simulink library "targets_stateflow_algorithms"  (Simulink 7.6)
settings: Solver=ode45  SolverMode=SingleTasking  StartTime=0.0  StopTime=10.0  RelTol=1e-3
values from neighbouring files (symbols this model uses):
  A1 = [1 -0.740818220682]    [targets_fsysdat.mat]
  A2 = [1 -0.740818220682]    [targets_fsysdat.mat]
  B1 = [8.76963147833 -8.51044969901]    [targets_fsysdat.mat]
  B2 = [0 0.259181779318]    [targets_fsysdat.mat]
  DISABLED = 3    [targets_fsysdat.mat]
  hys = 25    [targets_fsysdat.mat]
  Ki = 0.012    [targets_fsysdat.mat]
  LOW = 1    [targets_fsysdat.mat]
  max_ego = 1.2    [targets_fsysdat.mat]
  max_press = 1    [targets_fsysdat.mat]
  max_speed = 628    [targets_fsysdat.mat]
  max_throt = 90    [targets_fsysdat.mat]
  min_press = 0.0078    [targets_fsysdat.mat]
  min_throt = 3    [targets_fsysdat.mat]
  press = [0.05 0.1 0.15 0.2 0.25 0.3 0.35 0.4 0.45 0.5 0.55 0.6 ... (19 elements, 1x19)]    [targets_fsysdat.mat]
  PressEst = [0.806253176324 0.553142316929 0.37151500209 0.277667903103 0.220198954207 0.181288665766 0.153200000489 0.115431020872 0.0913067476324 0.0746519188607 0.0625231108324 0.0533383634277 ... (306 elements, 18x17)]    [targets_fsysdat.mat]
  pumpCon = [-0.0556348 -0.0022828 0.0256932 0.0435188 0.0562692 0.0661194857143 0.0741572 0.08697 0.0972452 0.106070342857 0.1139892 0.121303866667 ... (342 elements, 18x19)]    [targets_fsysdat.mat]
  RICH = 2    [targets_fsysdat.mat]
  SpeedEst = [471.837839721 550.80940091 777.559313277 1080.9243499 1418.36795322 1769.7468768 2125.37309264 2480.20345067 2831.37796793 3177.14006959 3516.32917143 4064.90417867 ... (323 elements, 17x19)]    [targets_fsysdat.mat]
  ThrotEst = [0 0 0 0 0 0 0 0 0 0 0 0 ... (342 elements, 18x19)]    [targets_fsysdat.mat]
  zero_thresh = 250    [targets_fsysdat.mat]
undefined symbols (not defined in the file or in its folder): fixpt_evenspace_cleanup
libraries: simulink x2, fixpt_lib_4 x1
settings Model: Creator=The MathWorks Inc.

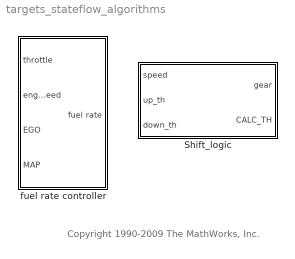
== system targets_stateflow_algorithms ==
  note: Copyright 1990-2009 The MathWorks, Inc.
  Shift_logic : Stateflow chart  TreatAsAtomicUnit=on
  fuel rate controller : Subsystem

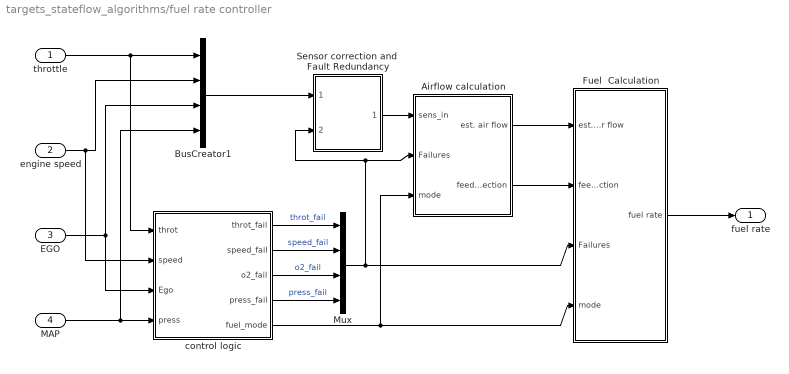
== system targets_stateflow_algorithms/fuel rate controller ==
  throttle : Inport
  engine speed : Inport  Port=2
  EGO : Inport  Port=3
  MAP : Inport  Port=4
  Airflow calculation : Subsystem
  BusCreator1 : BusCreator
  Fuel  Calculation : Subsystem
  Mux : Mux
  Sensor correction and  Fault Redundancy : Subsystem
  control logic : Stateflow chart  Description=Stateflow diagram to determine control system operating mode  TreatAsAtomicUnit=on
  fuel rate : Outport  InitialOutput=0
  wires:
  control logic/4(press_fail) -> Mux/4  "press_fail"
  control logic/3(o2_fail) -> Mux/3  "o2_fail"
  control logic/2(speed_fail) -> Mux/2  "speed_fail"
  control logic/1(throt_fail) -> Mux/1  "throt_fail"
  Mux/1 -> Fuel  Calculation/3(Failures), Airflow calculation/2(Failures), Sensor correction and  Fault Redundancy/2(Failures)
  Sensor correction and  Fault Redundancy/1(Corrected) -> Airflow calculation/1(sens_in)
  Airflow calculation/1(est. air flow) -> Fuel  Calculation/1(est. air flow)
  Fuel  Calculation/1(fuel rate) -> fuel rate/1
  Airflow calculation/2(feedback correction) -> Fuel  Calculation/2(feedback correction)
  control logic/5(fuel_mode) -> Fuel  Calculation/4(mode), Airflow calculation/3(mode)
  BusCreator1/1 -> Sensor correction and  Fault Redundancy/1(Sensors)
  throttle/1 -> control logic/1(throt), BusCreator1/1
  engine speed/1 -> control logic/2(speed), BusCreator1/2
  EGO/1 -> control logic/3(Ego), BusCreator1/3
  MAP/1 -> control logic/4(press), BusCreator1/4

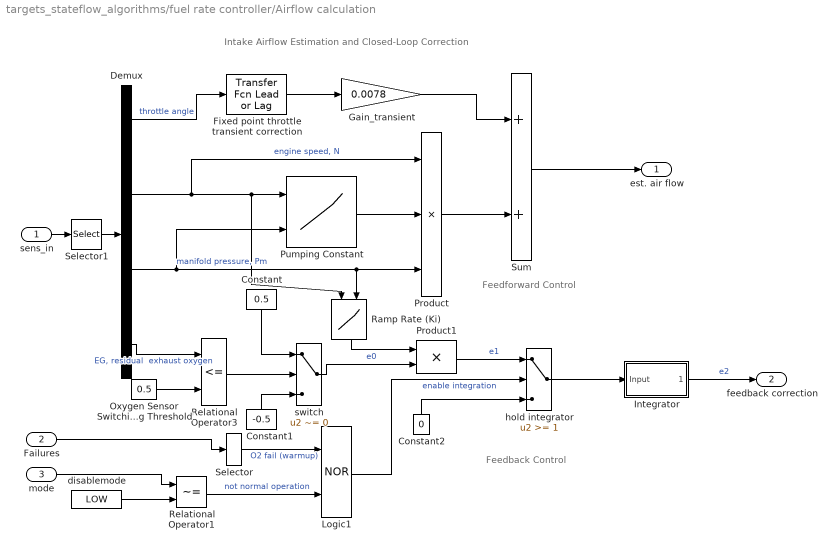
== system targets_stateflow_algorithms/fuel rate controller/Airflow calculation ==
  note: Feedforward Control
  note: Feedback Control
  note: Intake Airflow Estimation and Closed-Loop Correction
  sens_in : Inport
  Failures : Inport  Port=2
  mode : Inport  Port=3
  Constant : Constant  Value=0.5  OutDataTypeStr=fixdt(1,16,8)
  Constant1 : Constant  Value=-0.5  OutDataTypeStr=Inherit: Inherit via back propagation
  Constant2 : Constant  Value=0  OutDataTypeStr=Inherit: Inherit via back propagation
  Demux : Demux
  Fixed point throttle transient correction : simulink/Discrete/Transfer Fcn Lead or Lag  SystemSampleTime=-1  PoleZ=0.8  ZeroZ=1  ICPrevOutput=0.0  ICPrevInput=0.0  DoSatur=off
  Gain_transient : Gain  Gain=0.0078  OutDataTypeStr=fixdt(1,16,8)  SaturateOnIntegerOverflow=on  ParamDataTypeStr=Inherit: Same as input
  Integrator : Subsystem  Description=REQ: PM=30deg, GM=6db
      mask Display: disp('T/(Z-1)')
  Logic1 : Logic  Operator=NOR
  Oxygen Sensor Switching Threshold : Constant  Value=0.5  OutDataTypeStr=Inherit: Inherit via back propagation
  Product : Product  Inputs=3  OutDataTypeStr=fixdt(1,16,8)  SaturateOnIntegerOverflow=on
  Product1 : Product  SaturateOnIntegerOverflow=on  InputSameDT=on  OutDataTypeStr=Inherit: Same as first input
  Pumping Constant : Lookup2D  RowIndex=SpeedVect  ColumnIndex=fixpt_evenspace_cleanup(press,sfix(16),2^-14)  Table=pumpCon  LookUpMeth=Interpolation-Use End Values  OutDataTypeStr=fixdt(1,16,16)  SaturateOnIntegerOverflow=on
  Ramp Rate (Ki) : Lookup2D  RowIndex=[100:100:500]  ColumnIndex=fixpt_evenspace_cleanup([0:0.2:1],sfix(16),2^-14)  Table=[1:5]'*[1:6]*Ki  LookUpMeth=Interpolation-Use End Values  OutDataTypeStr=fixdt(1,16,8)  SaturateOnIntegerOverflow=on
  Relational Operator1 : RelationalOperator  Operator=~=  InputSameDT=on
  Relational Operator3 : RelationalOperator  Operator=<=  InputSameDT=on
  Selector : Selector  InputPortWidth=4  IndexOptions=Index vector (dialog)  Indices=3  OutputSizes=1
  Selector1 : Selector  InputPortWidth=4  IndexOptions=Index vector (dialog)  Indices=[1 2 4 3]  OutputSizes=1
  Sum : Sum  Inputs=2  SaturateOnIntegerOverflow=on  InputSameDT=on  OutDataTypeStr=Inherit: Same as first input
  disablemode : Constant  Value=LOW
  hold integrator : Switch  Threshold=1  SaturateOnIntegerOverflow=on  InputSameDT=on
  switch : Switch  Criteria=u2 ~= 0  Threshold=1  OutDataTypeStr=Inherit: Inherit via back propagation  SaturateOnIntegerOverflow=on  InputSameDT=on
  est. air flow : Outport  InitialOutput=0
  feedback correction : Outport  Port=2  InitialOutput=0
  wires:
  Gain_transient/1 -> Sum/1
  Fixed point throttle transient correction/1 -> Gain_transient/1
  Integrator/1(Output) -> feedback correction/1  "e2"
  Sum/1 -> est. air flow/1
  Constant1/1 -> switch/3
  Relational Operator3/1 -> switch/2
  switch/1 -> Product1/2  "e0"
  Logic1/1 -> hold integrator/2  "enable integration"
  hold integrator/1 -> Integrator/1(Input)
  Product1/1 -> hold integrator/1  "e1"
  Constant2/1 -> hold integrator/3
  Ramp Rate (Ki)/1 -> Product1/1
  Constant/1 -> switch/1
  Oxygen Sensor Switching Threshold/1 -> Relational Operator3/2
  Demux/4 -> Relational Operator3/1  "EG, residual  exhaust oxygen"
  Relational Operator1/1 -> Logic1/2  "not normal operation"
  disablemode/1 -> Relational Operator1/2
  Failures/1 -> Selector/1
  Selector/1 -> Logic1/1  "O2 fail (warmup)"
  Demux/1 -> Fixed point throttle transient correction/1  "throttle angle"
  Selector1/1 -> Demux/1
  Demux/2 -> Product/1, Ramp Rate (Ki)/1, Pumping Constant/1  "engine speed, N"
  Demux/3 -> Pumping Constant/2, Product/3, Ramp Rate (Ki)/2  "manifold pressure, Pm"
  Product/1 -> Sum/2
  Pumping Constant/1 -> Product/2
  sens_in/1 -> Selector1/1
  mode/1 -> Relational Operator1/1

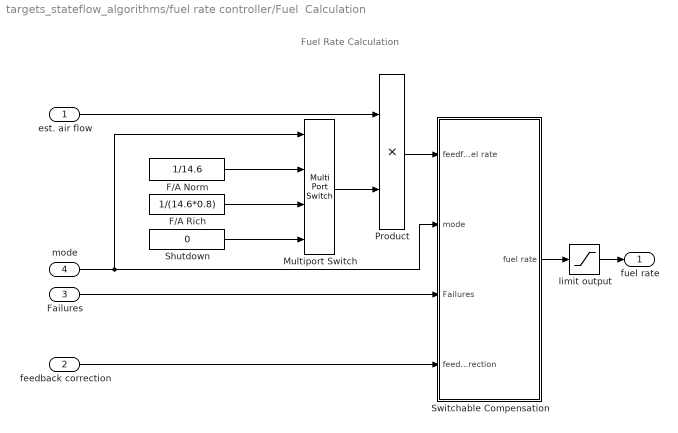
== system targets_stateflow_algorithms/fuel rate controller/Fuel  Calculation ==
  note: Fuel Rate Calculation
  est. air flow : Inport
  feedback correction : Inport  Port=2
  Failures : Inport  Port=3
  mode : Inport  Port=4
  F/A Norm : Constant  Value=1/14.6  OutDataTypeStr=fixdt(1,16,8)
  F/A Rich : Constant  Value=1/(14.6*0.8)  OutDataTypeStr=Inherit: Inherit via back propagation
  Multiport Switch : MultiPortSwitch  zeroidx=off  SaturateOnIntegerOverflow=on  InputSameDT=on
  Product : Product  OutDataTypeStr=fixdt(1,16,12)  SaturateOnIntegerOverflow=on  InputSameDT=on
  Shutdown : Constant  Value=0  OutDataTypeStr=Inherit: Inherit via back propagation
  Switchable Compensation : Subsystem
  limit output : Saturate  UpperLimit=100  LowerLimit=0
  fuel rate : Outport  InitialOutput=0
  wires:
  Switchable Compensation/1(fuel rate) -> limit output/1
  Product/1 -> Switchable Compensation/1(feedforward fuel rate)
  Failures/1 -> Switchable Compensation/3(Failures)
  mode/1 -> Multiport Switch/1, Switchable Compensation/2(mode)
  Multiport Switch/1 -> Product/2
  est. air flow/1 -> Product/1
  F/A Norm/1 -> Multiport Switch/2
  F/A Rich/1 -> Multiport Switch/3
  Shutdown/1 -> Multiport Switch/4
  feedback correction/1 -> Switchable Compensation/4(feedback correction)
  limit output/1 -> fuel rate/1

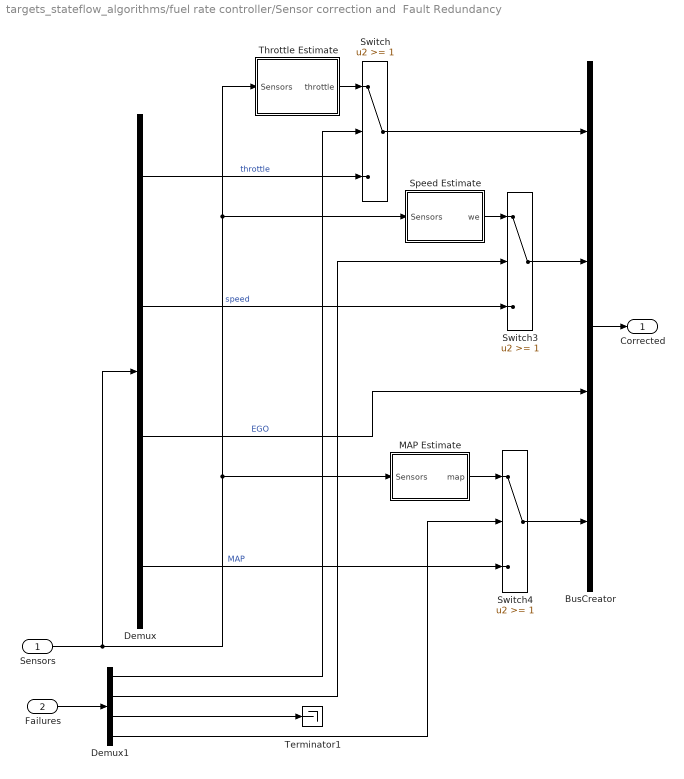
== system targets_stateflow_algorithms/fuel rate controller/Sensor correction and  Fault Redundancy ==
  Sensors : Inport
  Failures : Inport  Port=2
  BusCreator : BusCreator
  Demux : Demux
  Demux1 : Demux
  MAP Estimate : Subsystem  TreatAsAtomicUnit=on
  Speed Estimate : Subsystem  TreatAsAtomicUnit=on
  Switch : Switch  Threshold=1  SaturateOnIntegerOverflow=on  InputSameDT=on
  Switch3 : Switch  Threshold=1  SaturateOnIntegerOverflow=on  InputSameDT=on
  Switch4 : Switch  Threshold=1  SaturateOnIntegerOverflow=on
  Terminator1 : Terminator
  Throttle Estimate : Subsystem  TreatAsAtomicUnit=on
  Corrected : Outport  InitialOutput=0
  wires:
  BusCreator/1 -> Corrected/1
  Demux/3 -> BusCreator/3  "EGO"
  Switch/1 -> BusCreator/1
  Failures/1 -> Demux1/1
  Demux/1 -> Switch/3  "throttle"
  Throttle Estimate/1(throttle) -> Switch/1
  Demux1/3 -> Terminator1/1
  Demux1/1 -> Switch/2
  Switch3/1 -> BusCreator/2
  Demux/2 -> Switch3/3  "speed"
  Speed Estimate/1(we) -> Switch3/1
  Demux1/2 -> Switch3/2
  Demux1/4 -> Switch4/2
  Switch4/1 -> BusCreator/4
  Demux/4 -> Switch4/3  "MAP"
  MAP Estimate/1(map) -> Switch4/1
  Sensors/1 -> MAP Estimate/1(Sensors), Speed Estimate/1(Sensors), Throttle Estimate/1(Sensors), Demux/1

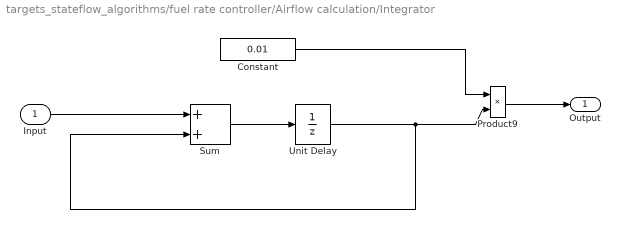
== system targets_stateflow_algorithms/fuel rate controller/Airflow calculation/Integrator ==
  Input : Inport
  Constant : Constant  Value=0.01  OutDataTypeStr=fixdt(1,16,12)
  Product9 : Product  SaturateOnIntegerOverflow=on  OutDataTypeStr=Inherit: Same as first input
  Sum : Sum  Tag=S16 2^-10  SaturateOnIntegerOverflow=on  InputSameDT=on  LockScale=on
  Unit Delay : UnitDelay  X0=-1  SampleTime=0.01
  Output : Outport
  wires:
  Input/1 -> Sum/1
  Sum/1 -> Unit Delay/1
  Product9/1 -> Output/1
  Constant/1 -> Product9/1
  Unit Delay/1 -> Sum/2, Product9/2

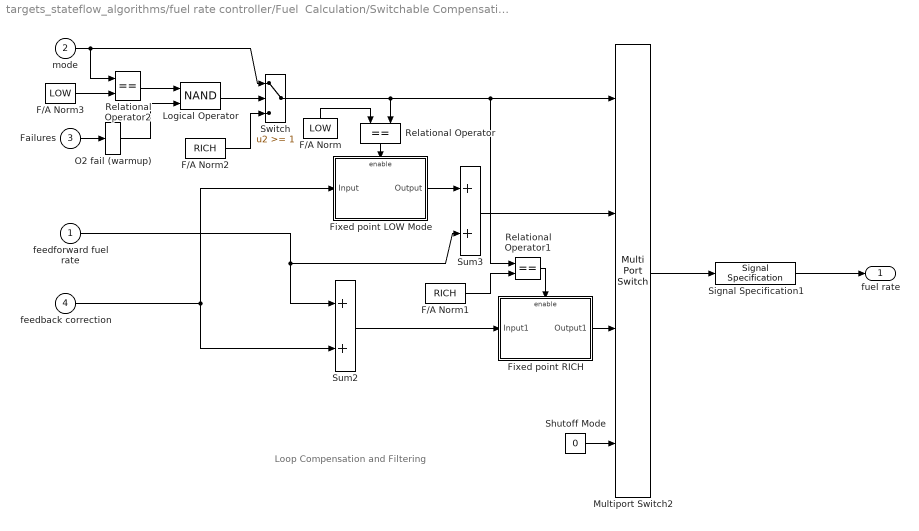
== system targets_stateflow_algorithms/fuel rate controller/Fuel  Calculation/Switchable Compensation ==
  note: Loop Compensation and Filtering
  feedforward fuel rate : Inport
  mode : Inport  Port=2
  Failures : Inport  Port=3
  feedback correction : Inport  Port=4
  F/A Norm : Constant  Value=LOW
  F/A Norm1 : Constant  Value=RICH
  F/A Norm2 : Constant  Value=RICH
  F/A Norm3 : Constant  Value=LOW
  Fixed point LOW Mode : Subsystem  TreatAsAtomicUnit=on  mask(enabled discrete-time transfer function){num=B1, den=A1, u0=-0.01, y0=-0.01, Ts=0.01}
      mask prompts: num "numerator polynomial"; den "denominator polynomial"; u0 "initial input"; y0 "initial output"; Ts "sample time"
      mask Display: dpoly(num,den,'z')
  Fixed point RICH : Subsystem  TreatAsAtomicUnit=on  mask(enabled discrete-time transfer function){num=B2, den=A2, u0=1.6, y0=1.6, Ts=0.01}
      mask prompts: num "numerator polynomial"; den "denominator polynomial"; u0 "initial input"; y0 "initial output"; Ts "sample time"
      mask Display: dpoly(num,den,'z')
  Logical Operator : Logic  Operator=NAND
  Multiport Switch2 : MultiPortSwitch  zeroidx=off  SaturateOnIntegerOverflow=on  InputSameDT=on
  O2 fail (warmup) : Selector  InputPortWidth=4  IndexOptions=Index vector (dialog)  Indices=3  OutputSizes=1
  Relational Operator : RelationalOperator  Operator===  InputSameDT=on
  Relational Operator1 : RelationalOperator  Operator===  InputSameDT=on
  Relational Operator2 : RelationalOperator  Operator===  InputSameDT=on
  Shutoff Mode : Constant  Value=0  OutDataTypeStr=Inherit: Inherit via back propagation
  Signal Specification1 : SignalSpecification  SampleTime=0.01
  Sum2 : Sum  OutDataTypeStr=fixdt(1,16,8)  SaturateOnIntegerOverflow=on  InputSameDT=on
  Sum3 : Sum  SaturateOnIntegerOverflow=on  OutDataTypeStr=Inherit: Same as first input
  Switch : Switch  Threshold=1  SaturateOnIntegerOverflow=on  InputSameDT=on
  fuel rate : Outport  InitialOutput=0
  wires:
  Fixed point LOW Mode/1(Output) -> Sum3/1
  Fixed point RICH/1(Output1) -> Multiport Switch2/3
  Signal Specification1/1 -> fuel rate/1
  O2 fail (warmup)/1 -> Logical Operator/2
  Failures/1 -> O2 fail (warmup)/1
  Relational Operator2/1 -> Logical Operator/1
  F/A Norm3/1 -> Relational Operator2/2
  mode/1 -> Relational Operator2/1, Switch/1
  Logical Operator/1 -> Switch/2
  F/A Norm2/1 -> Switch/3
  F/A Norm/1 -> Relational Operator/1
  Switch/1 -> Relational Operator/2, Multiport Switch2/1, Relational Operator1/1
  Multiport Switch2/1 -> Signal Specification1/1
  Relational Operator/1 -> Fixed point LOW Mode/Enable
  Relational Operator1/1 -> Fixed point RICH/Enable
  F/A Norm1/1 -> Relational Operator1/2
  Shutoff Mode/1 -> Multiport Switch2/4
  Sum2/1 -> Fixed point RICH/1(Input1)
  Sum3/1 -> Multiport Switch2/2
  feedback correction/1 -> Fixed point LOW Mode/1(Input), Sum2/2
  feedforward fuel rate/1 -> Sum2/1, Sum3/2

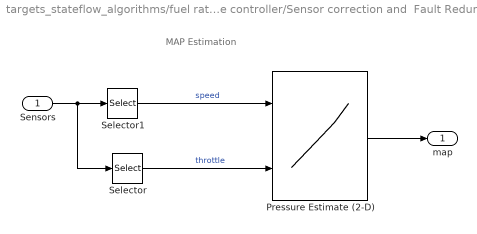
== system targets_stateflow_algorithms/fuel rate controller/Sensor correction and  Fault Redundancy/MAP Estimate ==
  note: MAP Estimation
  Sensors : Inport
  Pressure Estimate (2-D) : Lookup2D  RowIndex=SpeedVect  ColumnIndex=ThrotVect  Table=PressEst  LookUpMeth=Interpolation-Use End Values  OutDataTypeStr=fixdt(1,16,14)  SaturateOnIntegerOverflow=on
  Selector : Selector  InputPortWidth=4  IndexOptions=Index vector (dialog)  Indices=1  OutputSizes=1
  Selector1 : Selector  InputPortWidth=4  IndexOptions=Index vector (dialog)  Indices=2  OutputSizes=1
  map : Outport  InitialOutput=0
  wires:
  Pressure Estimate (2-D)/1 -> map/1
  Selector/1 -> Pressure Estimate (2-D)/2  "throttle"
  Selector1/1 -> Pressure Estimate (2-D)/1  "speed"
  Sensors/1 -> Selector/1, Selector1/1

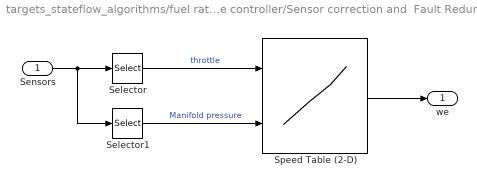
== system targets_stateflow_algorithms/fuel rate controller/Sensor correction and  Fault Redundancy/Speed Estimate ==
  Sensors : Inport
  Selector : Selector  InputPortWidth=4  IndexOptions=Index vector (dialog)  Indices=1  OutputSizes=1
  Selector1 : Selector  InputPortWidth=4  IndexOptions=Index vector (dialog)  Indices=4  OutputSizes=1
  Speed Table (2-D) : Lookup2D  RowIndex=ThrotVect  ColumnIndex=fixpt_evenspace_cleanup(press,sfix(16),2^-14)  Table=SpeedEst  LookUpMeth=Interpolation-Use End Values  OutDataTypeStr=fixdt(1,16,1)  SaturateOnIntegerOverflow=on
  we : Outport  InitialOutput=0
  wires:
  Selector1/1 -> Speed Table (2-D)/2  "Manifold pressure"
  Selector/1 -> Speed Table (2-D)/1  "throttle"
  Sensors/1 -> Selector/1, Selector1/1
  Speed Table (2-D)/1 -> we/1

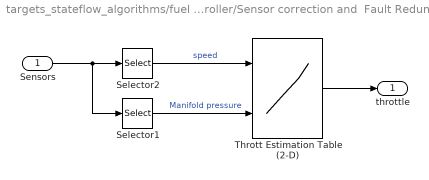
== system targets_stateflow_algorithms/fuel rate controller/Sensor correction and  Fault Redundancy/Throttle Estimate ==
  Sensors : Inport
  Selector1 : Selector  InputPortWidth=4  IndexOptions=Index vector (dialog)  Indices=4  OutputSizes=1
  Selector2 : Selector  InputPortWidth=4  IndexOptions=Index vector (dialog)  Indices=2  OutputSizes=1
  Thrott Estimation Table (2-D) : Lookup2D  RowIndex=SpeedVect  ColumnIndex=fixpt_evenspace_cleanup(press,sfix(16),2^-14)  Table=ThrotEst  LookUpMeth=Interpolation-Use End Values  OutDataTypeStr=fixdt(1,16,5)  SaturateOnIntegerOverflow=on
  throttle : Outport  InitialOutput=0
  wires:
  Thrott Estimation Table (2-D)/1 -> throttle/1
  Selector1/1 -> Thrott Estimation Table (2-D)/2  "Manifold pressure"
  Selector2/1 -> Thrott Estimation Table (2-D)/1  "speed"
  Sensors/1 -> Selector1/1, Selector2/1

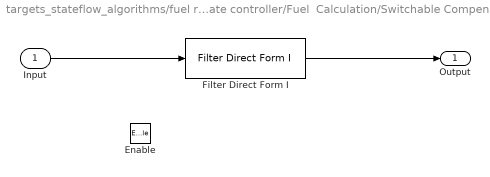
== system targets_stateflow_algorithms/fuel rate controller/Fuel  Calculation/Switchable Compensation/Fixed point LOW Mode ==
  Input : Inport
  Enable : EnablePort  StatesWhenEnabling=reset
  Filter Direct Form I : fixpt_lib_4/Filters/Filter Direct Form I  SystemSampleTime=-1  NumCoefVec=B1  DenCoefVec=A1(2)  ICPrevOutput=0.0  ICPrevInput=0.0  DoSatur=off
  Output : Outport
  wires:
  Filter Direct Form I/1 -> Output/1
  Input/1 -> Filter Direct Form I/1

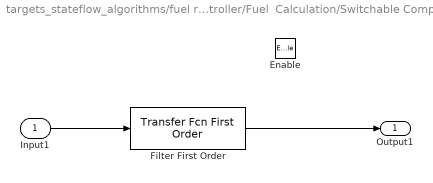
== system targets_stateflow_algorithms/fuel rate controller/Fuel  Calculation/Switchable Compensation/Fixed point RICH ==
  Input1 : Inport
  Enable : EnablePort  StatesWhenEnabling=reset
  Filter First Order : simulink/Discrete/Transfer Fcn First Order  SystemSampleTime=-1  PoleZ=-den(2)  ICPrevOutput=y0  DoSatur=off
  Output1 : Outport
  wires:
  Filter First Order/1 -> Output1/1
  Input1/1 -> Filter First Order/1

== stateflow chart fuel rate controller/control logic ==
  settings: updateMethod=DISCRETE  sampleTime=0.01
  state O2 [parallel]
    settings: executionOrder=1  description=This state determines the validity of the exhaust gas oxygen sensor (EGO) data.
    state fail
      entry: o2_fail = 1;
      settings: description=The EGO sensor has failed.
    state warmup
      entry: o2_fail = 1;
      during: warmup_clk++;
      settings: description=The EGO sensor must come up to temperature before its data is reliable.
    state normal
      entry: o2_fail = 0;
      settings: description=Normal EGO sensor operation gives a reliable indication of excess oxygen in the exhaust gas, from which air/fuel mixture can be inferred.
    O2.fail -> O2.normal : [Ego < max_ego] /
        | Fail.DEC
    O2.normal -> O2.fail : [Ego > max_ego]/
        | Fail.INC
      settings: description=The failure condition is indicated by excessive output voltage.
    (default) -> warmup
    warmup -> O2.normal : [warmup_clk>480]
      settings: description=It is assumed that the time o2_t_thresh is sufficient for the sensor to warm up to operational temperature.
  state Pressure [parallel]
    settings: executionOrder=2  description=This state assesses the validity of the manifold absolute pressure (MAP) sensor.
    state press_norm
      entry:  press_fail = 0;
      settings: description=The manifold pressure sensor gives a reliable indication of absolute pressure (MAP).
    state press_fail
      entry: press_fail = 1;
      settings: description=The pressure sensor (manifold, or MAP) no longer produces reliable data.
    press_norm -> press_fail : [press > max_press | press < min_press]
        | /Fail.INC
    (default) -> press_norm
    press_fail -> press_norm : [press > min_press & press < max_press] /
        | Fail.DEC
  state Throttle [parallel]
    settings: executionOrder=3  description=This state determines the validity of the throttle sensor signal.
    state normal
      entry: throt_fail = 0;
      settings: description=The throttle sensor gives a reliable indication of the angle of the throttle plate.
    state fail
      entry: throt_fail = 1;
      settings: description=Signal levels indicate that the throttle sensor data is no longer valid.
    Throttle.normal -> Throttle.fail : [throt> max_throt | throt < min_throt]/
        | Fail.INC
      settings: description=A failure is indicated by data which is outside the expected range, typically due to an open or short circuit.
    (default) -> Throttle.normal
    Throttle.fail -> Throttle.normal : [throt >  min_throt & throt < max_throt]
        | / Fail.DEC
  state Speed [parallel]
    settings: executionOrder=4  description="This state infers the validity of the speed sensor data.  A failure is indicated by the presence of manifold vacuum at zero speed."
    state normal
      entry: speed_fail = 0;
      settings: description=The speed sensor data accurately represents the engine speed.
    state fail
      entry: speed_fail = 1;
      settings: description=The engine speed data is no longer available.
    Speed.normal -> Speed.fail : [speed==0 & press < zero_thresh]/
        | Fail.INC
      settings: description="Loss of a reliable speed sensor signal will indicate zero speed.  This is deemed invalid when the manifold vacuum indicates otherwise."
    (default) -> Speed.normal
    Speed.fail -> Speed.normal : [speed > 0] /
        | Fail.DEC
  state Fail [parallel]
    settings: executionOrder=5  description=This state maintains a count of the number of sensors in failure mode.
    state Multi
      settings: description=This state represents any of the conditions in which more than one sensor is in failure mode.
      state Three
        settings: description=Three of the engine sensors have failed.
      state Four
        settings: description=All four of the engine sensors have failed.
      state Two
        settings: description=Two of the engine sensors have failed.
      Three -> Four [order 1] : INC
      Two -> Three [order 2] : INC
      Four -> Three : DEC
      Three -> Two [order 2] : DEC
    state One
      settings: description=One of the engine sensors has failed.
    state None
      settings: description=Zero failures; all sensors are operational.
    (default) -> None
    None -> One : INC
    One -> Two [order 1] : INC
    Two -> One [order 1] : DEC
    One -> None [order 2] : DEC
  state Fueling_Mode [parallel]
    settings: executionOrder=6  description=This state interprets the other states in the chart to directly control the fueling mode.
    state Fuel_Disabled
      entry: fuel_mode = DISABLED;
      settings: description=The fuel is completely shut off while in this state.
      state Overspeed
        settings: description=The speed is dangerously high, so shut off the fuel.
      state Shutdown
        settings: description=Cut off system operation due to multiple sensor failures.
      Overspeed -> (junction 35) : [in(Speed.normal) & ...
          | speed < (max_speed - hys)]
      (junction 35) -> Shutdown [order 2] : [in(Fail.Multi)]
    state Running
      settings: description=The fuel is actively controlled while in this state.
      (history)
      state Low_Emissions
        entry: fuel_mode = LOW;
        (history)
        state Normal
          settings: description=All sensors are in correct operating modes, so effective closed-loop mixture control can be used.
        state Warmup
          settings: description="The sensors are all operational, but the oxygen (EGO) sensor is warming up.  We'll target a stoichiometric ratio, nonetheless, but won't close the loop around exhaust gas oxygen."
        (junction 36) -> Normal [order 2]
        Warmup -> (junction 36) : [in(O2.normal)]
      state Rich_Mixture
        entry: fuel_mode = RICH;
        settings: description=This mode enriches the mixture, lowering the air/fuel ratio.
        state Single_Failure
          settings: description=Continue uninterrupted engine operation, but with a richer mixture.
      Normal -> Single_Failure : [in(Fail.One)]
      Single_Failure -> Normal : [in(Fail.None)]
      (junction 36) -> Single_Failure [order 1] : [in(Fail.One)]
    Running -> Overspeed [order 2] : [ speed > max_speed ]
    (junction 35) -> Running [order 1] : [!in(Fail.Multi)]
    Running -> Shutdown [order 1] : enter(Fail.Multi)
    Shutdown -> Rich_Mixture : exit(Fail.Multi)
    (default) -> Warmup
  data: throt_fail output boolean; speed_fail output boolean; o2_fail output boolean; press_fail output boolean; throt input fixdt(1,16,5) [0..120]; speed input fixdt(1,16,1) [0..1000]; Ego input fixdt(1,16,7) [-5..12]; press input fixdt(1,16,7) [0..2]; fuel_mode output uint8 [1..3] =1; max_ego parameter fixdt(1,16,7) [0..12]; max_press parameter fixdt(1,16,7) [0..2]; min_press parameter fixdt(1,16,7) [0..2]; min_throt parameter fixdt(1,16,5) [0..120]; max_throt parameter fixdt(1,16,5) [0..120]; zero_thresh parameter fixdt(1,16,6) [0..500]; max_speed parameter fixdt(1,16,1) [0..1000]; hys parameter fixdt(1,16,5) [0..1000]; LOW parameter uint8; RICH parameter uint8; DISABLED parameter uint8; warmup_clk local uint16
  data throt settings: description=throttle plate angle
  data speed settings: description=engine angular velocity
  data Ego settings: description=Exhaust Gas Oxygen
  data press settings: description=Manifold Absolute Pressure (MAP)
  data fuel_mode settings: description=fuel control mode: LOW = stoichiometric mixture, RICH = rich mixture, DISABLED = shut down
  data max_ego settings: description=parameter represents the upper end of the EGO sensor range
  data max_press settings: description=parameter represents the upper limt of valid pressure readings
  data min_press settings: description=parameter for the lower end of the valid pressure sensor range
  data min_throt settings: description=minimum valid throttle angle
  data max_throt settings: description=parameter to indicate the maximum valid throttle angle reading
  data zero_thresh settings: description=minimum manifold pressure expected at zero speed
  data max_speed settings: description=parameter for the upper end of the safe engine speed range
  data hys settings: description=Hysteresis in the upper speed limit to avoid chatter at the threshold.
  data LOW settings: description="constant represents \"low emissions\" or stoichiometric fuel mixture mode"
  data RICH settings: description=constant represents rich fuel mixture mode
  data DISABLED settings: description=constant represents zero fuel mode
  events: DEC local EITHER_EDGE_EVENT; INC local EITHER_EDGE_EVENT

== stateflow chart Shift_logic ==
  settings: updateMethod=DISCRETE  sampleTime=0.04
  state gear_state [parallel]
    settings: executionOrder=1
    state fourth
      entry: gear = 4;
    state second
      entry: gear = 2;
    state third
      entry: gear = 3;
    state first
      entry: gear = 1;
    third -> fourth [order 1] : UP
    second -> third [order 1] : UP
    first -> second : UP
    (default) -> first
    fourth -> third : DOWN
    third -> second [order 2] : DOWN
    second -> first [order 2] : DOWN
  state selection_state [parallel]
    during: CALC_TH;
    settings: executionOrder=2
    state downshifting
    state upshifting
    state steady_state
    (default) -> steady_state
    steady_state -> upshifting [order 1] : [speed > up_th]
    steady_state -> downshifting [order 2] : [speed < down_th]
    upshifting -> steady_state [order 2] : [speed < up_th]
    downshifting -> steady_state [order 2] : [speed > down_th]
    downshifting -> steady_state [order 1] : after(TWAIT,tick)
        | [speed <= down_th]
        | {gear_state.DOWN}
    upshifting -> steady_state [order 1] : after(TWAIT,tick)
        | [speed >= up_th]
        | {gear_state.UP}
  data: speed input single; gear output uint8 [1..4]; TWAIT parameter uint8; up_th input single; down_th input single
  events: DOWN local EITHER_EDGE_EVENT; UP local EITHER_EDGE_EVENT; CALC_TH output FUNCTION_CALL_EVENT
